simulink model "totalSystem"  (R2019b)
settings: Solver=FixedStepAuto  StartTime=0.0  StopTime=10.0  FixedStep=0.001  RelTol=1e-3
values from neighbouring files (symbols this model uses):
  ballPosInit = [0;0;0;0]    [init.m]    (also in init2.m)
  C_v = 16.5    [init.m]    (also in init2.m)
  g = 9.81    [init.m]    (also in init2.m)
  I0 = (m_p+3*m_m)*g/(3*K)    (= 0.37278)    [init.m]    (also in init2.m)
  I_b = m_b*r_b^2    (= 8.664e-06)    [init.m]    (also in init2.m)
  I_p = m_p*0.04^2/12    (= 0.00012)    [init.m]    (also in init2.m)
  K = 11    [init.m]    (also in init2.m)
  m_b = 0.024    [init.m]    (also in init2.m)
  m_m = 0.118    [init.m]    (also in init2.m)
  m_p = 0.9    [init.m]    (also in init2.m)
  motorPlateInit = [0;0;0;0;0;0.32]    [init.m]    (also in init2.m)
  r = 0.17    [init.m]    (also in init2.m)
  r_b = 0.019    [init.m]    (also in init2.m)
settings Model: Creator=chukh  LastModifiedBy=chukh

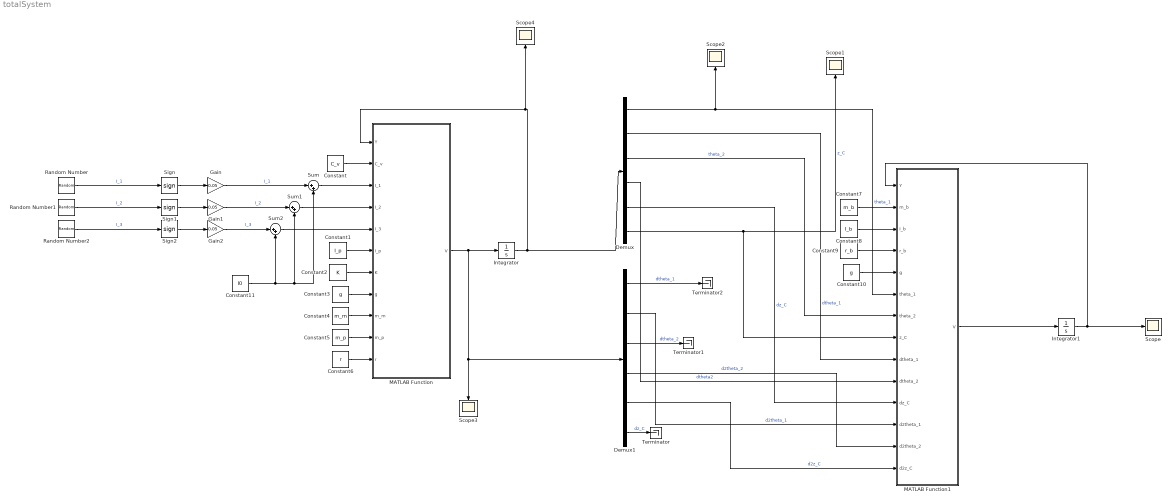
== system totalSystem ==
  Constant : Constant  Value=C_v
  Constant1 : Constant  Value=I_p
  Constant10 : Constant  Value=g
  Constant11 : Constant  Value=I0
  Constant2 : Constant  Value=K
  Constant3 : Constant  Value=g
  Constant4 : Constant  Value=m_m
  Constant5 : Constant  Value=m_p
  Constant6 : Constant  Value=r
  Constant7 : Constant  Value=m_b
  Constant8 : Constant  Value=I_b
  Constant9 : Constant  Value=r_b
  Demux : Demux  Outputs=6
  Demux1 : Demux  Outputs=6
  Gain : Gain  Gain=0.05
  Gain1 : Gain  Gain=0.05
  Gain2 : Gain  Gain=0.05
  Integrator : Integrator  InitialCondition=motorPlateInit
  Integrator1 : Integrator  InitialCondition=ballPosInit
  MATLAB Function : MATLAB Function  TreatAsAtomicUnit=on
  MATLAB Function1 : MATLAB Function  TreatAsAtomicUnit=on
  Random Number : RandomNumber  Seed=13  SampleTime=0.001
  Random Number1 : RandomNumber  Seed=23  SampleTime=0.001
  Random Number2 : RandomNumber  Seed=47  SampleTime=0.001
  Scope{,1..4} (5 alike) : Scope
  Sign : Signum
  Sign1 : Signum
  Sign2 : Signum
  Sum : Sum  Inputs=|++
  Sum1 : Sum  Inputs=|++
  Sum2 : Sum  Inputs=|++
  Terminator : Terminator
  Terminator1 : Terminator
  Terminator2 : Terminator
  wires:
  Demux/6 -> Scope1/1, MATLAB Function1/8(z_C)  "z_C"
  Demux/2 -> MATLAB Function1/9(dtheta_1)  "dtheta_1"
  Demux/3 -> MATLAB Function1/7(theta_2)  "theta_2"
  Demux/4 -> MATLAB Function1/10(dtheta_2)  "dtheta2"
  Demux/5 -> MATLAB Function1/11(dz_C)  "dz_C"
  Demux1/6 -> Terminator/1  "dz_C"
  Demux1/1 -> Terminator2/1  "dtheta_1"
  Demux1/2 -> MATLAB Function1/12(d2theta_1)  "d2theta_1"
  Demux1/3 -> Terminator1/1  "dtheta_2"
  Demux1/4 -> MATLAB Function1/13(d2theta_2)  "d2theta_2"
  Demux1/5 -> MATLAB Function1/14(d2z_C)  "d2z_C"
  MATLAB Function1/1(V) -> Integrator1/1
  Integrator1/1 -> Scope/1, MATLAB Function1/1(Y)
  Constant7/1 -> MATLAB Function1/2(m_b)
  Constant8/1 -> MATLAB Function1/3(I_b)
  Constant9/1 -> MATLAB Function1/4(r_b)
  Constant10/1 -> MATLAB Function1/5(g)
  Demux/1 -> Scope2/1, MATLAB Function1/6(theta_1)  "theta_1"
  Constant5/1 -> MATLAB Function/10(m_p)
  MATLAB Function/1(V) -> Demux1/1, Scope3/1, Integrator/1
  Random Number/1 -> Sign/1  "I_1"
  Constant4/1 -> MATLAB Function/9(m_m)
  Integrator/1 -> Demux/1, Scope4/1, MATLAB Function/1(Y)
  Constant/1 -> MATLAB Function/2(C_v)
  Constant2/1 -> MATLAB Function/7(K)
  Random Number2/1 -> Sign2/1  "I_3"
  Constant6/1 -> MATLAB Function/11(r)
  Constant1/1 -> MATLAB Function/6(I_p)
  Random Number1/1 -> Sign1/1  "I_2"
  Constant3/1 -> MATLAB Function/8(g)
  Sign/1 -> Gain/1
  Sign1/1 -> Gain1/1
  Sign2/1 -> Gain2/1
  Sum1/1 -> MATLAB Function/4(I_2)
  Gain1/1 -> Sum1/1  "I_2"
  Gain2/1 -> Sum2/1  "I_3"
  Sum2/1 -> MATLAB Function/5(I_3)
  Constant11/1 -> Sum/2, Sum1/2, Sum2/2
  Gain/1 -> Sum/1  "I_1"
  Sum/1 -> MATLAB Function/3(I_1)

== matlab function totalSystem/MATLAB Function1 ==
  data: Y input; V output; m_b input; I_b input; r_b input; g input; theta_1 input; theta_2 input; z_C input; dtheta_1 input; dtheta_2 input; dz_C input; d2theta_1 input; d2theta_2 input; d2z_C input
function V = ballOnPlateODE(Y,m_b,I_b,r_b,g,theta_1,theta_2,z_C,dtheta_1,dtheta_2,dz_C,d2theta_1,d2theta_2,d2z_C)
%BALLONPLATEODE
%    V = BALLONPLATEODE(Y,M_B,I_B,R_B,G,THETA_1,THETA_2,Z_C,DTHETA_1,DTHETA_2,DZ_C,D2THETA_1,D2THETA_2,D2Z_C)

%    This function was generated by the Symbolic Math Toolbox version 8.4.
%    16-May-2021 00:03:52

%matrix([[xf], [Dxf], [yf], [Dyf]])
t2 = cos(theta_1);
t3 = cos(theta_2);
t4 = sin(theta_1);
t5 = sin(theta_2);
t6 = Y(1);
t7 = Y(2);
t8 = Y(3);
t9 = Y(4);
t10 = dtheta_1.^2;
t11 = dtheta_2.^2;
t12 = r_b.^2;
t13 = r_b.^3;
t14 = t2.^2;
t15 = t2.^3;
t16 = t3.^2;
t18 = t3.^3;
t20 = t4.^2;
t21 = t4.^3;
t22 = t5.^2;
t24 = t5.^3;
t28 = m_b.*t12;
t17 = t14.^2;
t19 = t16.^2;
t23 = t20.^2;
t25 = t22.^2;
t26 = 1.0./t14;
t27 = 1.0./t16;
t29 = I_b+t28;
t30 = t14+t20;
t31 = 1.0./t29;
t32 = 1.0./t30;
V = [t7;(t26.*t27.*t31.*t32.*(I_b.*d2theta_2.*r_b.*t15.*t18+I_b.*r_b.*t11.*t15.*t24.*2.0-I_b.*t6.*t11.*t17.*t19-I_b.*t6.*t11.*t17.*t25.*2.0+d2z_C.*t5.*t17.*t18.*t28+g.*t5.*t17.*t18.*t28+m_b.*t11.*t13.*t15.*t24.*2.0-t6.*t11.*t17.*t25.*t28.*2.0+d2theta_2.*m_b.*t3.*t13.*t15.*t22+d2theta_1.*t5.*t8.*t16.*t17.*t28-d2theta_2.*t5.*t6.*t17.*t18.*t28-d2theta_2.*t3.*t6.*t17.*t24.*t28+dtheta_1.*t5.*t9.*t16.*t17.*t28.*2.0-dtheta_2.*t5.*t7.*t17.*t18.*t28.*2.0+dtheta_1.*t5.*t9.*t17.*t18.*t28-dtheta_2.*t3.*t7.*t17.*t24.*t28.*2.0+m_b.*t5.*t10.*t13.*t15.*t16.*2.0+m_b.*t5.*t11.*t13.*t15.*t16+t4.*t8.*t11.*t15.*t24.*t28.*2.0-t6.*t10.*t16.*t17.*t22.*t28-t6.*t11.*t16.*t17.*t22.*t28.*2.0+I_b.*dtheta_1.*dtheta_2.*r_b.*t18.*t21.*2.0+I_b.*dtheta_1.*dtheta_2.*t8.*t17.*t18.*2.0-I_b.*dtheta_1.*dtheta_2.*t8.*t17.*t19+I_b.*dtheta_1.*dtheta_2.*t8.*t18.*t23.*2.0+I_b.*d2theta_2.*r_b.*t2.*t18.*t20+I_b.*d2theta_2.*r_b.*t3.*t15.*t22+I_b.*d2theta_1.*t5.*t8.*t16.*t17+I_b.*d2theta_2.*t4.*t8.*t15.*t18-I_b.*d2theta_2.*t5.*t6.*t17.*t18-I_b.*d2theta_1.*t5.*t8.*t17.*t18+I_b.*d2theta_2.*t2.*t8.*t18.*t21-I_b.*d2theta_2.*t3.*t6.*t17.*t24+I_b.*dtheta_1.*t5.*t9.*t16.*t17.*2.0+I_b.*dtheta_2.*t4.*t9.*t15.*t18.*2.0-I_b.*dtheta_2.*t5.*t7.*t17.*t18.*2.0-I_b.*dtheta_1.*t5.*t9.*t17.*t18+I_b.*dtheta_2.*t2.*t9.*t18.*t21.*2.0-I_b.*dtheta_2.*t3.*t7.*t17.*t24.*2.0+I_b.*r_b.*t5.*t10.*t15.*t16+I_b.*r_b.*t5.*t11.*t15.*t16.*2.0+I_b.*r_b.*t2.*t11.*t20.*t24.*2.0+I_b.*t4.*t8.*t11.*t15.*t24.*2.0+I_b.*t2.*t8.*t11.*t21.*t24.*2.0-I_b.*t6.*t11.*t14.*t19.*t20-I_b.*t6.*t11.*t16.*t17.*t22.*3.0-I_b.*t6.*t11.*t14.*t20.*t25.*2.0+I_b.*dtheta_1.*dtheta_2.*r_b.*t4.*t14.*t18.*2.0-I_b.*dtheta_1.*dtheta_2.*r_b.*t4.*t14.*t22+I_b.*dtheta_1.*dtheta_2.*r_b.*t3.*t21.*t22.*2.0+I_b.*dtheta_1.*dtheta_2.*t4.*t6.*t15.*t24+I_b.*dtheta_1.*dtheta_2.*t3.*t8.*t17.*t22.*2.0+I_b.*dtheta_1.*dtheta_2.*t3.*t8.*t22.*t23.*2.0+I_b.*dtheta_1.*dtheta_2.*t8.*t14.*t18.*t20.*4.0-I_b.*dtheta_1.*dtheta_2.*t8.*t14.*t19.*t20-I_b.*dtheta_1.*dtheta_2.*t8.*t14.*t20.*t22-I_b.*d2theta_1.*r_b.*t3.*t4.*t5.*t14+I_b.*d2theta_1.*r_b.*t4.*t5.*t14.*t16+I_b.*d2theta_2.*r_b.*t2.*t3.*t20.*t22+I_b.*d2theta_1.*t3.*t4.*t6.*t15.*t22-I_b.*d2theta_1.*t3.*t5.*t8.*t14.*t20+I_b.*d2theta_2.*t3.*t4.*t8.*t15.*t22+I_b.*d2theta_2.*t2.*t3.*t8.*t21.*t22+I_b.*d2theta_1.*t5.*t8.*t14.*t16.*t20-I_b.*d2theta_2.*t5.*t6.*t14.*t18.*t20-I_b.*d2theta_2.*t3.*t6.*t14.*t20.*t24+I_b.*dtheta_1.*t3.*t4.*t7.*t15.*t22-I_b.*dtheta_1.*t3.*t5.*t9.*t14.*t20+I_b.*dtheta_2.*t3.*t4.*t9.*t15.*t22.*2.0+I_b.*dtheta_2.*t2.*t3.*t9.*t21.*t22.*2.0+I_b.*dtheta_1.*t5.*t9.*t14.*t16.*t20.*2.0-I_b.*dtheta_2.*t5.*t7.*t14.*t18.*t20.*2.0-I_b.*dtheta_2.*t3.*t7.*t14.*t20.*t24.*2.0+I_b.*r_b.*t2.*t5.*t10.*t16.*t20+I_b.*r_b.*t2.*t5.*t11.*t16.*t20.*2.0-I_b.*t3.*t4.*t5.*t8.*t10.*t15+I_b.*t4.*t5.*t8.*t10.*t15.*t16+I_b.*t4.*t5.*t8.*t11.*t15.*t16.*2.0+I_b.*t4.*t5.*t8.*t10.*t15.*t18+I_b.*t2.*t5.*t8.*t10.*t16.*t21+I_b.*t2.*t5.*t8.*t11.*t16.*t21.*2.0-I_b.*t3.*t6.*t10.*t14.*t20.*t22-I_b.*t6.*t11.*t14.*t16.*t20.*t22.*3.0+dtheta_1.*dtheta_2.*m_b.*t4.*t13.*t14.*t22-dtheta_1.*dtheta_2.*t4.*t6.*t15.*t24.*t28+dtheta_1.*dtheta_2.*t3.*t8.*t17.*t22.*t28.*2.0+dtheta_1.*dtheta_2.*t8.*t14.*t20.*t22.*t28+d2theta_1.*m_b.*t4.*t5.*t13.*t14.*t16+d2theta_2.*t3.*t4.*t8.*t15.*t22.*t28+d2theta_1.*t5.*t8.*t14.*t16.*t20.*t28-dtheta_1.*t3.*t4.*t7.*t15.*t22.*t28+dtheta_1.*t3.*t5.*t9.*t14.*t20.*t28+dtheta_2.*t3.*t4.*t9.*t15.*t22.*t28.*2.0+dtheta_1.*t5.*t9.*t14.*t16.*t20.*t28.*2.0+m_b.*t2.*t3.*t5.*t10.*t13.*t20.*2.0+m_b.*t2.*t5.*t10.*t13.*t16.*t20+t3.*t4.*t5.*t8.*t10.*t15.*t28+t2.*t3.*t5.*t8.*t10.*t21.*t28.*2.0+t4.*t5.*t8.*t10.*t15.*t16.*t28+t4.*t5.*t8.*t11.*t15.*t16.*t28+t4.*t5.*t8.*t10.*t15.*t18.*t28+t2.*t5.*t8.*t10.*t16.*t21.*t28-t3.*t6.*t10.*t14.*t20.*t22.*t28+I_b.*dtheta_1.*dtheta_2.*r_b.*t3.*t4.*t14.*t22.*2.0+I_b.*dtheta_1.*dtheta_2.*t4.*t5.*t6.*t15.*t16+I_b.*dtheta_1.*dtheta_2.*t3.*t8.*t14.*t20.*t22.*4.0-I_b.*dtheta_1.*dtheta_2.*t8.*t14.*t16.*t20.*t22+dtheta_1.*dtheta_2.*m_b.*t3.*t4.*t13.*t14.*t22.*2.0+dtheta_1.*dtheta_2.*t3.*t8.*t14.*t20.*t22.*t28.*2.0))./(t16+t22);t9;-t26.*t27.*t31.*t32.*(I_b.*d2theta_1.*r_b.*t3.*t15+I_b.*r_b.*t10.*t16.*t21.*2.0+I_b.*t3.*t8.*t10.*t17+I_b.*t8.*t10.*t16.*t17-I_b.*t8.*t10.*t17.*t18+I_b.*t8.*t10.*t16.*t23.*2.0+d2z_C.*t4.*t15.*t18.*t28+g.*t4.*t15.*t18.*t28+m_b.*t10.*t13.*t16.*t21.*2.0-t3.*t8.*t10.*t17.*t28+t8.*t10.*t16.*t17.*t28.*2.0-t8.*t10.*t17.*t18.*t28+t8.*t10.*t16.*t23.*t28.*2.0+d2theta_1.*m_b.*t2.*t13.*t16.*t20+d2theta_1.*t4.*t8.*t15.*t16.*t28-d2theta_2.*t4.*t6.*t15.*t18.*t28+d2theta_1.*t2.*t8.*t16.*t21.*t28-dtheta_1.*t3.*t4.*t9.*t15.*t28+dtheta_1.*t3.*t5.*t7.*t17.*t28+dtheta_1.*t4.*t9.*t15.*t16.*t28.*2.0-dtheta_2.*t4.*t7.*t15.*t18.*t28.*2.0+dtheta_1.*t4.*t9.*t15.*t18.*t28+dtheta_1.*t2.*t9.*t16.*t21.*t28.*2.0-m_b.*t3.*t4.*t10.*t13.*t14.*2.0+m_b.*t4.*t10.*t13.*t14.*t16.*3.0+m_b.*t4.*t11.*t13.*t14.*t16+m_b.*t4.*t11.*t13.*t14.*t22.*2.0-t3.*t8.*t10.*t14.*t20.*t28.*2.0-t4.*t6.*t11.*t15.*t24.*t28.*2.0+t8.*t10.*t14.*t16.*t20.*t28.*4.0+t8.*t11.*t14.*t16.*t20.*t28+t8.*t11.*t14.*t20.*t22.*t28.*2.0+I_b.*dtheta_1.*dtheta_2.*r_b.*t5.*t15-I_b.*dtheta_1.*dtheta_2.*t6.*t16.*t17-I_b.*dtheta_1.*dtheta_2.*t6.*t17.*t22+I_b.*d2theta_1.*r_b.*t2.*t16.*t20+I_b.*d2theta_1.*t3.*t4.*t8.*t15-I_b.*d2theta_1.*t3.*t5.*t6.*t17+I_b.*d2theta_1.*t4.*t8.*t15.*t16-I_b.*d2theta_1.*t4.*t8.*t15.*t18+I_b.*d2theta_1.*t2.*t8.*t16.*t21+I_b.*dtheta_1.*t3.*t4.*t9.*t15-I_b.*dtheta_1.*t3.*t5.*t7.*t17+I_b.*dtheta_1.*t4.*t9.*t15.*t16.*2.0-I_b.*dtheta_1.*t4.*t9.*t15.*t18+I_b.*dtheta_1.*t2.*t9.*t16.*t21.*2.0+I_b.*r_b.*t4.*t10.*t14.*t16.*2.0+I_b.*t8.*t10.*t14.*t16.*t20.*3.0-dtheta_1.*dtheta_2.*m_b.*t5.*t13.*t15+dtheta_1.*dtheta_2.*t6.*t17.*t22.*t28+I_b.*dtheta_1.*dtheta_2.*t4.*t5.*t8.*t15+I_b.*t3.*t4.*t5.*t6.*t10.*t15-dtheta_1.*dtheta_2.*t4.*t5.*t8.*t15.*t28+d2theta_2.*m_b.*t3.*t4.*t5.*t13.*t14-d2theta_2.*t3.*t4.*t6.*t15.*t22.*t28+d2theta_2.*t3.*t5.*t8.*t14.*t20.*t28-dtheta_2.*t3.*t4.*t7.*t15.*t22.*t28.*2.0+dtheta_2.*t3.*t5.*t9.*t14.*t20.*t28.*2.0+t3.*t4.*t5.*t6.*t10.*t15.*t28-t4.*t5.*t6.*t10.*t15.*t16.*t28-t4.*t5.*t6.*t11.*t15.*t16.*t28.*2.0+I_b.*dtheta_1.*dtheta_2.*t4.*t5.*t8.*t15.*t16+dtheta_1.*dtheta_2.*m_b.*t2.*t3.*t5.*t13.*t20.*2.0+dtheta_1.*dtheta_2.*t3.*t4.*t5.*t8.*t15.*t28.*2.0+dtheta_1.*dtheta_2.*t2.*t3.*t5.*t8.*t21.*t28.*2.0)];

== matlab function totalSystem/MATLAB Function ==
  data: V output; Y input; C_v input; I_1 input; I_2 input; I_3 input; I_p input; K input; g input; m_m input; m_p input; r input
function V = motorPlateODE(Y,C_v,I_1,I_2,I_3,I_p,K,g,m_m,m_p,r)
%MOTORPLATEODE
%    V = MOTORPLATEODE(T,Y,C_V,I_1,I_2,I_3,I_P,K,G,M_M,M_P,R)

%    This function was generated by the Symbolic Math Toolbox version 8.4.
%    18-May-2021 19:45:09

%matrix([[theta_1f], [omega_1f], [theta_2f], [omega_2f], [dz_Cf], [z_Cf]])
t2 = I_p.^2;
t3 = Y(1);
t4 = Y(2);
t5 = Y(3);
t6 = Y(4);
t7 = Y(5);
t8 = m_m.^2;
t9 = r.^2;
t10 = r.^3;
t19 = sqrt(3.0);
t11 = t9.^2;
t12 = cos(t3);
t13 = cos(t5);
t14 = sin(t3);
t15 = sin(t5);
t16 = t2.*4.0;
t17 = t4.^2;
t18 = t6.^2;
t20 = t12.^2;
t21 = t12.^3;
t22 = t13.^2;
t23 = t13.^3;
t25 = t14.^2;
t26 = t15.^2;
t24 = t22.^2;
t27 = I_p.*m_m.*t9.*t22.*6.0;
t29 = I_p.*m_m.*t9.*t25.*t26.*6.0;
t28 = t20.*t27;
t30 = t8.*t11.*t20.*t24.*9.0;
t31 = t16+t27+t28+t29+t30;
t32 = 1.0./t31;
V = [t4;t32.*(t12.*t14.*t17.*t27+t12.*t14.*t18.*t27+t8.*t11.*t12.*t14.*t17.*t24.*9.0+t8.*t11.*t12.*t14.*t18.*t24.*9.0-C_v.*I_p.*t4.*t9.*t20.*t22.*6.0-C_v.*m_m.*t4.*t11.*t20.*t24.*9.0+I_2.*I_p.*K.*r.*t12.*t13.*t19.*2.0-I_3.*I_p.*K.*r.*t12.*t13.*t19.*2.0+I_2.*K.*m_m.*t10.*t12.*t19.*t23.*3.0-I_3.*K.*m_m.*t10.*t12.*t19.*t23.*3.0+t4.*t6.*t8.*t11.*t15.*t20.*t23.*1.8e+1+t8.*t11.*t12.*t14.*t18.*t22.*t26.*1.8e+1-t8.*t11.*t14.*t18.*t21.*t22.*t26.*9.0-t8.*t11.*t12.*t14.^3.*t18.*t22.*t26.*9.0-t4.*t6.*t8.*t11.*t13.*t15.^3.*t20.*t25.*9.0+C_v.*I_p.*t6.*t9.*t12.*t13.*t14.*t15.*6.0-I_1.*K.*m_m.*t10.*t12.*t14.*t15.*t22.*6.0+I_2.*K.*m_m.*t10.*t12.*t14.*t15.*t22.*3.0+I_3.*K.*m_m.*t10.*t12.*t14.*t15.*t22.*3.0+I_p.*m_m.*t4.*t6.*t9.*t13.*t15.*t20.*1.2e+1+t4.*t6.*t8.*t11.*t13.*t15.*t20.*t25.*9.0-t4.*t6.*t8.*t11.*t15.*t20.*t23.*t25.*9.0);t6;-r.*t32.*(I_1.*I_p.*K.*t13.*4.0-I_2.*I_p.*K.*t13.*2.0-I_3.*I_p.*K.*t13.*2.0+C_v.*I_p.*r.*t6.*t22.*6.0-t8.*t10.*t15.*t18.*t20.*t23.*1.8e+1+t8.*t10.*t15.*t18.*t20.^2.*t23.*9.0+I_2.*I_p.*K.*t14.*t15.*t19.*2.0-I_3.*I_p.*K.*t14.*t15.*t19.*2.0+C_v.*I_p.*r.*t6.*t25.*t26.*6.0+I_1.*K.*m_m.*t9.*t20.*t23.*6.0-I_2.*K.*m_m.*t9.*t20.*t23.*3.0-I_3.*K.*m_m.*t9.*t20.*t23.*3.0+C_v.*m_m.*t6.*t10.*t20.*t24.*9.0-I_p.*m_m.*r.*t13.*t15.*t18.*1.2e+1-I_p.*m_m.*r.*t4.*t6.*t12.*t14.*6.0+I_p.*m_m.*r.*t13.*t15.*t18.*t20.*6.0+I_p.*m_m.*r.*t13.*t15.*t17.*t25.*6.0+I_p.*m_m.*r.*t13.*t15.*t18.*t25.*1.2e+1-t4.*t6.*t8.*t10.*t14.*t21.*t22.*9.0+t4.*t6.*t8.*t10.*t14.*t21.*t24.*9.0+t8.*t10.*t15.*t18.*t20.*t23.*t25.*9.0-C_v.*I_p.*r.*t4.*t12.*t13.*t14.*t15.*6.0+I_p.*m_m.*r.*t4.*t6.*t12.*t14.*t22.*6.0+I_p.*m_m.*r.*t4.*t6.*t12.*t14.*t26.*1.8e+1+t4.*t6.*t8.*t10.*t14.*t21.*t22.*t26.*9.0);-(C_v.*t7.*3.0+g.*m_m.*3.0+g.*m_p-I_1.*K-I_2.*K-I_3.*K)./(m_m.*3.0+m_p);t7];
